simulink model "simulacion_signal"  (R2021b)
settings: Solver=VariableStepAuto  StartTime=0.0  StopTime=15  RelTol=1e-3
settings Model: Creator=Alumno103  LastModifiedBy=Alumno103

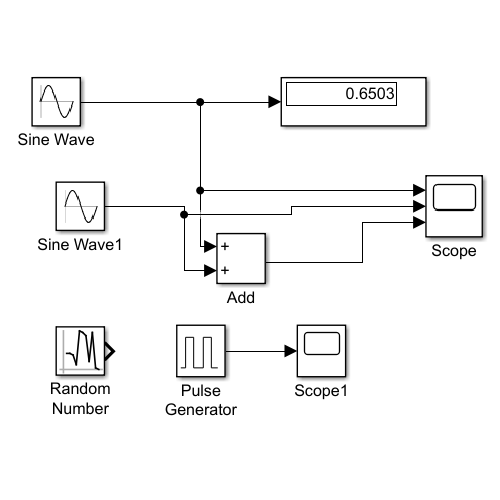
[thumbnail: Simulink's stored preview of the top-level diagram]
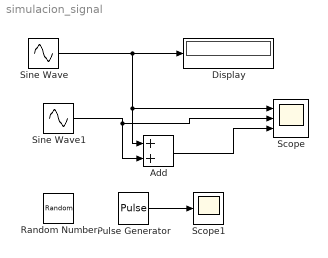
== system simulacion_signal ==
  Add : Sum
  Display : Display
  Pulse Generator : DiscretePulseGenerator  PulseType=Time based  PulseWidth=5
  Random Number : RandomNumber  SampleTime=0.1
  Scope : Scope  NumInputPorts=3
  Scope1 : Scope
  Sine Wave : Sin  SampleTime=0
  Sine Wave1 : Sin  Amplitude=2  Frequency=2  SampleTime=0
  wires:
  Sine Wave/1 -> Add/1, Scope/1, Display/1
  Sine Wave1/1 -> Add/2, Scope/2
  Add/1 -> Scope/3
  Pulse Generator/1 -> Scope1/1
